simulink model "MdXXIsPosChk"  (R2024b)
settings: Solver=FixedStepDiscrete  StartTime=0.0  StopTime=10.0  FixedStep=0.01  RelTol=1e-3
libraries: simulink x35
(part 2 of 2)

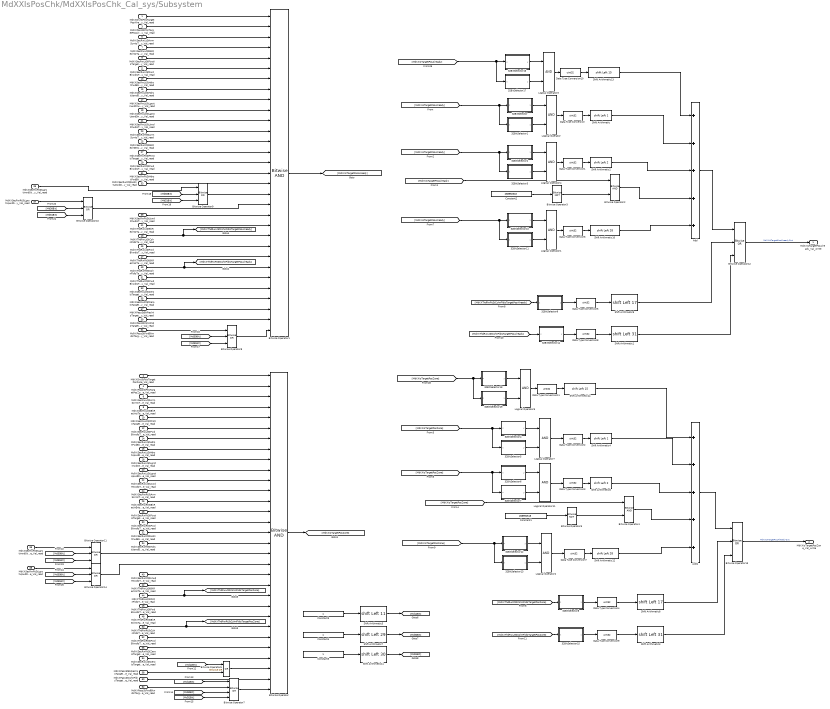
== system MdXXIsPosChk/MdXXIsPosChk_Cal_sys/Subsystem ==
  MdXXDrvStFtIsTargetPosAlready_Val_read : Inport
  MdXXDrvStFtIsTargetPosZone_Val_read : Inport  Port=2
  MdXXPassStFtIsTargetPosAlready_Val_read : Inport  Port=3
  MdXXPassStFtIsTargetPosZone_Val_read : Inport  Port=4
  MdXXSecRwLtStArmScrnIsTargetPosAlready_Val_read : Inport  Port=5
  MdXXSecRwLtStArmScrnIsTargetPosZone_Val_read : Inport  Port=6
  MdXXSecRwLtStBkReclnIsTargetPosAlready_Val_read : Inport  Port=7
  MdXXSecRwLtStBkReclnIsTargetPosZone_Val_read : Inport  Port=8
  MdXXSecRwLtStFtrstIsTargetPosAlready_Val_read : Inport  Port=9
  MdXXSecRwLtStFtrstIsTargetPosZone_Val_read : Inport  Port=10
  MdXXSecRwLtStFwdBkwdIsTargetPosAlready_Val_read : Inport  Port=11
  MdXXSecRwLtStFwdBkwdIsTargetPosZone_Val_read : Inport  Port=12
  MdXXSecRwLtStHdrstFwdBkwdIsTargetPosAlready_Val_read : Inport  Port=13
  MdXXSecRwLtStHdrstFwdBkwdIsTargetPosZone_Val_read : Inport  Port=14
  MdXXSecRwLtStHdrstUpwdDnwdIsTargetPosAlready_Val_read : Inport  Port=15
  MdXXSecRwLtStHdrstUpwdDnwdIsTargetPosZone_Val_read : Inport  Port=16
  MdXXSecRwLtStLgrstInwdOtwdIsTargetPosAlready_Val_read : Inport  Port=17
  MdXXSecRwLtStLgrstInwdOtwdIsTargetPosZone_Val_read : Inport  Port=18
  MdXXSecRwLtStLgrstUpwdDnwdIsTargetPosAlready_Val_read : Inport  Port=19
  MdXXSecRwLtStLgrstUpwdDnwdIsTargetPosZone_Val_read : Inport  Port=20
  MdXXSecRwLtStLtwdRtwdIsTargetPosAlready_Val_read : Inport  Port=21
  MdXXSecRwLtStLtwdRtwdIsTargetPosZone_Val_read : Inport  Port=22
  MdXXSecRwRtStArmScrnIsTargetPosAlready_Val_read : Inport  Port=23
  MdXXSecRwRtStArmScrnIsTargetPosZone_Val_read : Inport  Port=24
  MdXXSecRwRtStBkReclnEnIsTargetPosAlready_Val_read : Inport  Port=25
  MdXXSecRwRtStBkReclnEnIsTargetPosZone_Val_read : Inport  Port=26
  MdXXSecRwRtStFtrstIsTargetPosAlready_Val_read : Inport  Port=27
  MdXXSecRwRtStFtrstIsTargetPosZone_Val_read : Inport  Port=28
  MdXXSecRwRtStFwdBkwdIsTargetPosAlready_Val_read : Inport  Port=29
  MdXXSecRwRtStFwdBkwdIsTargetPosZone_Val_read : Inport  Port=30
  MdXXSecRwRtStHdrstFwdBkwdIsTargetPosAlready_Val_read : Inport  Port=31
  MdXXSecRwRtStHdrstFwdBkwdIsTargetPosZone_Val_read : Inport  Port=32
  MdXXSecRwRtStHdrstUpwdDnwdIsTargetPosAlready_Val_read : Inport  Port=33
  MdXXSecRwRtStHdrstUpwdDnwdIsTargetPosZone_Val_read : Inport  Port=34
  MdXXSecRwRtStLgrstInwdOtwdIsTargetPosAlready_Val_read : Inport  Port=35
  MdXXSecRwRtStLgrstInwdOtwdIsTargetPosZone_Val_read : Inport  Port=36
  MdXXSecRwRtStLgrstUpwdDnwdIsTargetPosAlready_Val_read : Inport  Port=37
  MdXXSecRwRtStLgrstUpwdDnwdIsTargetPosZone_Val_read : Inport  Port=38
  MdXXSecRwRtStLtwdRtwdIsTargetPosAlready_Val_read : Inport  Port=39
  MdXXSecRwRtStLtwdRtwdIsTargetPosZone_Val_read : Inport  Port=40
  MdXXThdRwLtStBkReclnIsTargetPosAlready_Val_read : Inport  Port=41
  MdXXThdRwLtStBkReclnIsTargetPosZone_Val_read : Inport  Port=42
  MdXXThdRwLtStCshnFldIsTargetPosAlready_Val_read : Inport  Port=43
  MdXXThdRwLtStCshnFldIsTargetPosZone_Val_read : Inport  Port=44
  MdXXThdRwLtStFwdBkwdIsTargetPosAlready_Val_read : Inport  Port=45
  MdXXThdRwLtStFwdBkwdIsTargetPosZone_Val_read : Inport  Port=46
  MdXXThdRwRtStBkReclnIsTargetPosAlready_Val_read : Inport  Port=47
  MdXXThdRwRtStBkReclnIsTargetPosZone_Val_read : Inport  Port=48
  MdXXThdRwRtStCshnFldIsTargetPosAlready_Val_read : Inport  Port=49
  MdXXThdRwRtStCshnFldIsTargetPosZone_Val_read : Inport  Port=50
  MdXXThdRwRtStFwdBkwdIsTargetPosAlready_Val_read : Inport  Port=51
  MdXXThdRwRtStFwdBkwdIsTargetPosZone_Val_read : Inport  Port=52
  MdXXSecRwLtStZeroIsTargetPosAlready_Val_read : Inport  Port=53
  MdXXSecRwLtStZeroIsTargetPosZone_Val_read : Inport  Port=54
  MdXXSecRwRtStZeroIsTargetPosAlready_Val_read : Inport  Port=55
  MdXXSecRwRtStZeroIsTargetPosZone_Val_read : Inport  Port=56
  MdXXPassStBkReclnIsTargetPosAlready_Val_read : Inport  Port=57
  MdXXPassStBkReclnIsTargetPosZone_Val_read : Inport  Port=58
  MdXXPassStCshnFldIsTargetPosAlready_Val_read : Inport  Port=59
  MdXXPassStCshnFldIsTargetPosZone_Val_read : Inport  Port=60
  MdXXPassStFwdBkwdIsTargetPosAlready_Val_read : Inport  Port=61
  MdXXPassStFwdBkwdIsTargetPosZone_Val_read : Inport  Port=62
  32BitSelector : Subsystem  mask(32 Bit Selector){BitNum=9}
      mask prompts: BitNum "Select Bit Number"
      mask help: Allows selection of a particular bit (0-31) out of a packed word up to 32 bits long. Output will be true if the bit number selected via the mask parameter is equal to one.
      mask TypeOptions BitNum: 0 | 1 | 2 | 3 | 4 | 5 | 6 | 7 | 8 | 9 | 10 | 11 | 12 | 13 | 14 | 15 | 16 | 17 | 18 | 19 | 20 | 21 | 22 | 23 | 24 | 25 | 26 | 27 | 28 | 29 | 30 | 31
      mask Display:
      | text(0.5, 0.8,'BIT','horizontalAlignment','center')
      | text(0.5, 0.5,'SELECTOR','horizontalAlignment','center')
      | text(0.5, 0.2,['-- Bit ',char(get_param(gcb,'BitNum')),' --'],'horizontalAlignment','center')
  32BitSelector1 : Subsystem  mask(32 Bit Selector){BitNum=11}
      mask prompts: BitNum "Select Bit Number"
      mask help: Allows selection of a particular bit (0-31) out of a packed word up to 32 bits long. Output will be true if the bit number selected via the mask parameter is equal to one.
      mask TypeOptions BitNum: 0 | 1 | 2 | 3 | 4 | 5 | 6 | 7 | 8 | 9 | 10 | 11 | 12 | 13 | 14 | 15 | 16 | 17 | 18 | 19 | 20 | 21 | 22 | 23 | 24 | 25 | 26 | 27 | 28 | 29 | 30 | 31
      mask Display:
      | text(0.5, 0.8,'BIT','horizontalAlignment','center')
      | text(0.5, 0.5,'SELECTOR','horizontalAlignment','center')
      | text(0.5, 0.2,['-- Bit ',char(get_param(gcb,'BitNum')),' --'],'horizontalAlignment','center')
  32BitSelector10 : Subsystem  mask(32 Bit Selector){BitNum=26}
      mask prompts: BitNum "Select Bit Number"
      mask help: Allows selection of a particular bit (0-31) out of a packed word up to 32 bits long. Output will be true if the bit number selected via the mask parameter is equal to one.
      mask TypeOptions BitNum: 0 | 1 | 2 | 3 | 4 | 5 | 6 | 7 | 8 | 9 | 10 | 11 | 12 | 13 | 14 | 15 | 16 | 17 | 18 | 19 | 20 | 21 | 22 | 23 | 24 | 25 | 26 | 27 | 28 | 29 | 30 | 31
      mask Display:
      | text(0.5, 0.8,'BIT','horizontalAlignment','center')
      | text(0.5, 0.5,'SELECTOR','horizontalAlignment','center')
      | text(0.5, 0.2,['-- Bit ',char(get_param(gcb,'BitNum')),' --'],'horizontalAlignment','center')
  32BitSelector11 : Subsystem  mask(32 Bit Selector){BitNum=27}
      mask prompts: BitNum "Select Bit Number"
      mask help: Allows selection of a particular bit (0-31) out of a packed word up to 32 bits long. Output will be true if the bit number selected via the mask parameter is equal to one.
      mask TypeOptions BitNum: 0 | 1 | 2 | 3 | 4 | 5 | 6 | 7 | 8 | 9 | 10 | 11 | 12 | 13 | 14 | 15 | 16 | 17 | 18 | 19 | 20 | 21 | 22 | 23 | 24 | 25 | 26 | 27 | 28 | 29 | 30 | 31
      mask Display:
      | text(0.5, 0.8,'BIT','horizontalAlignment','center')
      | text(0.5, 0.5,'SELECTOR','horizontalAlignment','center')
      | text(0.5, 0.2,['-- Bit ',char(get_param(gcb,'BitNum')),' --'],'horizontalAlignment','center')
  32BitSelector12 : Subsystem  mask(32 Bit Selector){BitNum=26}
      mask prompts: BitNum "Select Bit Number"
      mask help: Allows selection of a particular bit (0-31) out of a packed word up to 32 bits long. Output will be true if the bit number selected via the mask parameter is equal to one.
      mask TypeOptions BitNum: 0 | 1 | 2 | 3 | 4 | 5 | 6 | 7 | 8 | 9 | 10 | 11 | 12 | 13 | 14 | 15 | 16 | 17 | 18 | 19 | 20 | 21 | 22 | 23 | 24 | 25 | 26 | 27 | 28 | 29 | 30 | 31
      mask Display:
      | text(0.5, 0.8,'BIT','horizontalAlignment','center')
      | text(0.5, 0.5,'SELECTOR','horizontalAlignment','center')
      | text(0.5, 0.2,['-- Bit ',char(get_param(gcb,'BitNum')),' --'],'horizontalAlignment','center')
  32BitSelector13 : Subsystem  mask(32 Bit Selector){BitNum=27}
      mask prompts: BitNum "Select Bit Number"
      mask help: Allows selection of a particular bit (0-31) out of a packed word up to 32 bits long. Output will be true if the bit number selected via the mask parameter is equal to one.
      mask TypeOptions BitNum: 0 | 1 | 2 | 3 | 4 | 5 | 6 | 7 | 8 | 9 | 10 | 11 | 12 | 13 | 14 | 15 | 16 | 17 | 18 | 19 | 20 | 21 | 22 | 23 | 24 | 25 | 26 | 27 | 28 | 29 | 30 | 31
      mask Display:
      | text(0.5, 0.8,'BIT','horizontalAlignment','center')
      | text(0.5, 0.5,'SELECTOR','horizontalAlignment','center')
      | text(0.5, 0.2,['-- Bit ',char(get_param(gcb,'BitNum')),' --'],'horizontalAlignment','center')
  32BitSelector14 : Subsystem  mask(32 Bit Selector){BitNum=31}
      mask prompts: BitNum "Select Bit Number"
      mask help: Allows selection of a particular bit (0-31) out of a packed word up to 32 bits long. Output will be true if the bit number selected via the mask parameter is equal to one.
      mask TypeOptions BitNum: 0 | 1 | 2 | 3 | 4 | 5 | 6 | 7 | 8 | 9 | 10 | 11 | 12 | 13 | 14 | 15 | 16 | 17 | 18 | 19 | 20 | 21 | 22 | 23 | 24 | 25 | 26 | 27 | 28 | 29 | 30 | 31
      mask Display:
      | text(0.5, 0.8,'BIT','horizontalAlignment','center')
      | text(0.5, 0.5,'SELECTOR','horizontalAlignment','center')
      | text(0.5, 0.2,['-- Bit ',char(get_param(gcb,'BitNum')),' --'],'horizontalAlignment','center')
  32BitSelector15 : Subsystem  mask(32 Bit Selector){BitNum=31}
      mask prompts: BitNum "Select Bit Number"
      mask help: Allows selection of a particular bit (0-31) out of a packed word up to 32 bits long. Output will be true if the bit number selected via the mask parameter is equal to one.
      mask TypeOptions BitNum: 0 | 1 | 2 | 3 | 4 | 5 | 6 | 7 | 8 | 9 | 10 | 11 | 12 | 13 | 14 | 15 | 16 | 17 | 18 | 19 | 20 | 21 | 22 | 23 | 24 | 25 | 26 | 27 | 28 | 29 | 30 | 31
      mask Display:
      | text(0.5, 0.8,'BIT','horizontalAlignment','center')
      | text(0.5, 0.5,'SELECTOR','horizontalAlignment','center')
      | text(0.5, 0.2,['-- Bit ',char(get_param(gcb,'BitNum')),' --'],'horizontalAlignment','center')
  32BitSelector16 : Subsystem  mask(32 Bit Selector){BitNum=13}
      mask prompts: BitNum "Select Bit Number"
      mask help: Allows selection of a particular bit (0-31) out of a packed word up to 32 bits long. Output will be true if the bit number selected via the mask parameter is equal to one.
      mask TypeOptions BitNum: 0 | 1 | 2 | 3 | 4 | 5 | 6 | 7 | 8 | 9 | 10 | 11 | 12 | 13 | 14 | 15 | 16 | 17 | 18 | 19 | 20 | 21 | 22 | 23 | 24 | 25 | 26 | 27 | 28 | 29 | 30 | 31
      mask Display:
      | text(0.5, 0.8,'BIT','horizontalAlignment','center')
      | text(0.5, 0.5,'SELECTOR','horizontalAlignment','center')
      | text(0.5, 0.2,['-- Bit ',char(get_param(gcb,'BitNum')),' --'],'horizontalAlignment','center')
  32BitSelector17 : Subsystem  mask(32 Bit Selector){BitNum=14}
      mask prompts: BitNum "Select Bit Number"
      mask help: Allows selection of a particular bit (0-31) out of a packed word up to 32 bits long. Output will be true if the bit number selected via the mask parameter is equal to one.
      mask TypeOptions BitNum: 0 | 1 | 2 | 3 | 4 | 5 | 6 | 7 | 8 | 9 | 10 | 11 | 12 | 13 | 14 | 15 | 16 | 17 | 18 | 19 | 20 | 21 | 22 | 23 | 24 | 25 | 26 | 27 | 28 | 29 | 30 | 31
      mask Display:
      | text(0.5, 0.8,'BIT','horizontalAlignment','center')
      | text(0.5, 0.5,'SELECTOR','horizontalAlignment','center')
      | text(0.5, 0.2,['-- Bit ',char(get_param(gcb,'BitNum')),' --'],'horizontalAlignment','center')
  32BitSelector18 : Subsystem  mask(32 Bit Selector){BitNum=13}
      mask prompts: BitNum "Select Bit Number"
      mask help: Allows selection of a particular bit (0-31) out of a packed word up to 32 bits long. Output will be true if the bit number selected via the mask parameter is equal to one.
      mask TypeOptions BitNum: 0 | 1 | 2 | 3 | 4 | 5 | 6 | 7 | 8 | 9 | 10 | 11 | 12 | 13 | 14 | 15 | 16 | 17 | 18 | 19 | 20 | 21 | 22 | 23 | 24 | 25 | 26 | 27 | 28 | 29 | 30 | 31
      mask Display:
      | text(0.5, 0.8,'BIT','horizontalAlignment','center')
      | text(0.5, 0.5,'SELECTOR','horizontalAlignment','center')
      | text(0.5, 0.2,['-- Bit ',char(get_param(gcb,'BitNum')),' --'],'horizontalAlignment','center')
  32BitSelector19 : Subsystem  mask(32 Bit Selector){BitNum=14}
      mask prompts: BitNum "Select Bit Number"
      mask help: Allows selection of a particular bit (0-31) out of a packed word up to 32 bits long. Output will be true if the bit number selected via the mask parameter is equal to one.
      mask TypeOptions BitNum: 0 | 1 | 2 | 3 | 4 | 5 | 6 | 7 | 8 | 9 | 10 | 11 | 12 | 13 | 14 | 15 | 16 | 17 | 18 | 19 | 20 | 21 | 22 | 23 | 24 | 25 | 26 | 27 | 28 | 29 | 30 | 31
      mask Display:
      | text(0.5, 0.8,'BIT','horizontalAlignment','center')
      | text(0.5, 0.5,'SELECTOR','horizontalAlignment','center')
      | text(0.5, 0.2,['-- Bit ',char(get_param(gcb,'BitNum')),' --'],'horizontalAlignment','center')
  32BitSelector2 : Subsystem  mask(32 Bit Selector){BitNum=7}
      mask prompts: BitNum "Select Bit Number"
      mask help: Allows selection of a particular bit (0-31) out of a packed word up to 32 bits long. Output will be true if the bit number selected via the mask parameter is equal to one.
      mask TypeOptions BitNum: 0 | 1 | 2 | 3 | 4 | 5 | 6 | 7 | 8 | 9 | 10 | 11 | 12 | 13 | 14 | 15 | 16 | 17 | 18 | 19 | 20 | 21 | 22 | 23 | 24 | 25 | 26 | 27 | 28 | 29 | 30 | 31
      mask Display:
      | text(0.5, 0.8,'BIT','horizontalAlignment','center')
      | text(0.5, 0.5,'SELECTOR','horizontalAlignment','center')
      | text(0.5, 0.2,['-- Bit ',char(get_param(gcb,'BitNum')),' --'],'horizontalAlignment','center')
  32BitSelector3 : Subsystem  mask(32 Bit Selector){BitNum=8}
      mask prompts: BitNum "Select Bit Number"
      mask help: Allows selection of a particular bit (0-31) out of a packed word up to 32 bits long. Output will be true if the bit number selected via the mask parameter is equal to one.
      mask TypeOptions BitNum: 0 | 1 | 2 | 3 | 4 | 5 | 6 | 7 | 8 | 9 | 10 | 11 | 12 | 13 | 14 | 15 | 16 | 17 | 18 | 19 | 20 | 21 | 22 | 23 | 24 | 25 | 26 | 27 | 28 | 29 | 30 | 31
      mask Display:
      | text(0.5, 0.8,'BIT','horizontalAlignment','center')
      | text(0.5, 0.5,'SELECTOR','horizontalAlignment','center')
      | text(0.5, 0.2,['-- Bit ',char(get_param(gcb,'BitNum')),' --'],'horizontalAlignment','center')
  32BitSelector4 : Subsystem  mask(32 Bit Selector){BitNum=9}
      mask prompts: BitNum "Select Bit Number"
      mask help: Allows selection of a particular bit (0-31) out of a packed word up to 32 bits long. Output will be true if the bit number selected via the mask parameter is equal to one.
      mask TypeOptions BitNum: 0 | 1 | 2 | 3 | 4 | 5 | 6 | 7 | 8 | 9 | 10 | 11 | 12 | 13 | 14 | 15 | 16 | 17 | 18 | 19 | 20 | 21 | 22 | 23 | 24 | 25 | 26 | 27 | 28 | 29 | 30 | 31
      mask Display:
      | text(0.5, 0.8,'BIT','horizontalAlignment','center')
      | text(0.5, 0.5,'SELECTOR','horizontalAlignment','center')
      | text(0.5, 0.2,['-- Bit ',char(get_param(gcb,'BitNum')),' --'],'horizontalAlignment','center')
  32BitSelector5 : Subsystem  mask(32 Bit Selector){BitNum=11}
      mask prompts: BitNum "Select Bit Number"
      mask help: Allows selection of a particular bit (0-31) out of a packed word up to 32 bits long. Output will be true if the bit number selected via the mask parameter is equal to one.
      mask TypeOptions BitNum: 0 | 1 | 2 | 3 | 4 | 5 | 6 | 7 | 8 | 9 | 10 | 11 | 12 | 13 | 14 | 15 | 16 | 17 | 18 | 19 | 20 | 21 | 22 | 23 | 24 | 25 | 26 | 27 | 28 | 29 | 30 | 31
      mask Display:
      | text(0.5, 0.8,'BIT','horizontalAlignment','center')
      | text(0.5, 0.5,'SELECTOR','horizontalAlignment','center')
      | text(0.5, 0.2,['-- Bit ',char(get_param(gcb,'BitNum')),' --'],'horizontalAlignment','center')
  32BitSelector6 : Subsystem  mask(32 Bit Selector){BitNum=7}
      mask prompts: BitNum "Select Bit Number"
      mask help: Allows selection of a particular bit (0-31) out of a packed word up to 32 bits long. Output will be true if the bit number selected via the mask parameter is equal to one.
      mask TypeOptions BitNum: 0 | 1 | 2 | 3 | 4 | 5 | 6 | 7 | 8 | 9 | 10 | 11 | 12 | 13 | 14 | 15 | 16 | 17 | 18 | 19 | 20 | 21 | 22 | 23 | 24 | 25 | 26 | 27 | 28 | 29 | 30 | 31
      mask Display:
      | text(0.5, 0.8,'BIT','horizontalAlignment','center')
      | text(0.5, 0.5,'SELECTOR','horizontalAlignment','center')
      | text(0.5, 0.2,['-- Bit ',char(get_param(gcb,'BitNum')),' --'],'horizontalAlignment','center')
  32BitSelector7 : Subsystem  mask(32 Bit Selector){BitNum=8}
      mask prompts: BitNum "Select Bit Number"
      mask help: Allows selection of a particular bit (0-31) out of a packed word up to 32 bits long. Output will be true if the bit number selected via the mask parameter is equal to one.
      mask TypeOptions BitNum: 0 | 1 | 2 | 3 | 4 | 5 | 6 | 7 | 8 | 9 | 10 | 11 | 12 | 13 | 14 | 15 | 16 | 17 | 18 | 19 | 20 | 21 | 22 | 23 | 24 | 25 | 26 | 27 | 28 | 29 | 30 | 31
      mask Display:
      | text(0.5, 0.8,'BIT','horizontalAlignment','center')
      | text(0.5, 0.5,'SELECTOR','horizontalAlignment','center')
      | text(0.5, 0.2,['-- Bit ',char(get_param(gcb,'BitNum')),' --'],'horizontalAlignment','center')
  32BitSelector8 : Subsystem  mask(32 Bit Selector){BitNum=17}
      mask prompts: BitNum "Select Bit Number"
      mask help: Allows selection of a particular bit (0-31) out of a packed word up to 32 bits long. Output will be true if the bit number selected via the mask parameter is equal to one.
      mask TypeOptions BitNum: 0 | 1 | 2 | 3 | 4 | 5 | 6 | 7 | 8 | 9 | 10 | 11 | 12 | 13 | 14 | 15 | 16 | 17 | 18 | 19 | 20 | 21 | 22 | 23 | 24 | 25 | 26 | 27 | 28 | 29 | 30 | 31
      mask Display:
      | text(0.5, 0.8,'BIT','horizontalAlignment','center')
      | text(0.5, 0.5,'SELECTOR','horizontalAlignment','center')
      | text(0.5, 0.2,['-- Bit ',char(get_param(gcb,'BitNum')),' --'],'horizontalAlignment','center')
  32BitSelector9 : Subsystem  mask(32 Bit Selector){BitNum=17}
      mask prompts: BitNum "Select Bit Number"
      mask help: Allows selection of a particular bit (0-31) out of a packed word up to 32 bits long. Output will be true if the bit number selected via the mask parameter is equal to one.
      mask TypeOptions BitNum: 0 | 1 | 2 | 3 | 4 | 5 | 6 | 7 | 8 | 9 | 10 | 11 | 12 | 13 | 14 | 15 | 16 | 17 | 18 | 19 | 20 | 21 | 22 | 23 | 24 | 25 | 26 | 27 | 28 | 29 | 30 | 31
      mask Display:
      | text(0.5, 0.8,'BIT','horizontalAlignment','center')
      | text(0.5, 0.5,'SELECTOR','horizontalAlignment','center')
      | text(0.5, 0.2,['-- Bit ',char(get_param(gcb,'BitNum')),' --'],'horizontalAlignment','center')
  Add : Sum  Inputs=+++++  OutDataTypeStr=uint32
  Add1 : Sum  Inputs=+++++  AccumDataTypeStr=uint32
  Bitwise Operator : simulink/Logic and Bit Operations/Bitwise Operator  logicop=AND  UseBitMask=off  NumInputPorts=31  BitMask=bin2dec('11011001')  BitMaskRealWorld=Stored Integer
  Bitwise Operator1 : simulink/Logic and Bit Operations/Bitwise Operator  logicop=AND  UseBitMask=off  NumInputPorts=31  BitMask=bin2dec('11011001')  BitMaskRealWorld=Stored Integer
  Bitwise Operator{8..14} (7 alike) : simulink/Logic and Bit Operations/Bitwise Operator  logicop=OR  UseBitMask=off  NumInputPorts=3  BitMask=bin2dec('11011001')  BitMaskRealWorld=Stored Integer
  Bitwise Operator2 : simulink/Logic and Bit Operations/Bitwise Operator  logicop=AND  UseBitMask=off  NumInputPorts=2  BitMask=bin2dec('11011001')  BitMaskRealWorld=Stored Integer
  Bitwise Operator3 : simulink/Logic and Bit Operations/Bitwise Operator  logicop=NOT  UseBitMask=off  BitMask=bin2dec('11011001')  BitMaskRealWorld=Stored Integer
  Bitwise Operator4 : simulink/Logic and Bit Operations/Bitwise Operator  logicop=AND  UseBitMask=off  NumInputPorts=2  BitMask=bin2dec('11011001')  BitMaskRealWorld=Stored Integer
  Bitwise Operator5 : simulink/Logic and Bit Operations/Bitwise Operator  logicop=NOT  UseBitMask=off  BitMask=bin2dec('11011001')  BitMaskRealWorld=Stored Integer
  Bitwise Operator6 : simulink/Logic and Bit Operations/Bitwise Operator  logicop=OR  UseBitMask=off  NumInputPorts=2  BitMask=bin2dec('11011001')  BitMaskRealWorld=Stored Integer
  Bitwise Operator7 : simulink/Logic and Bit Operations/Bitwise Operator  logicop=OR  UseBitMask=off  NumInputPorts=4  BitMask=bin2dec('11011001')  BitMaskRealWorld=Stored Integer
  Constant1 : Constant  Value=268992518  OutDataTypeStr=uint32
  Constant2 : Constant  Value=268992518  OutDataTypeStr=uint32
  Constant3 : Constant  OutDataTypeStr=uint32
  Constant4 : Constant  OutDataTypeStr=uint32
  Constant5 : Constant  OutDataTypeStr=uint32
  Data Type Conversion{,1..11} (12 alike) : DataTypeConversion  OutDataTypeStr=uint32  SaturateOnIntegerOverflow=off  RndMeth=Floor
  Logical Operator{,1..5,7,11} (8 alike) : Logic  AllPortsSameDT=off  OutDataTypeStr=boolean
  Shift Arithmetic : ArithShift  BitShiftNumber=1  BitShiftDirection=Left
  Shift Arithmetic1 : ArithShift  BitShiftNumber=31  BitShiftDirection=Left
  Shift Arithmetic10 : ArithShift  BitShiftNumber=28  BitShiftDirection=Left
  Shift Arithmetic11 : ArithShift  BitShiftNumber=30  BitShiftDirection=Left
  Shift Arithmetic12 : ArithShift  BitShiftNumber=28  BitShiftDirection=Left
  Shift Arithmetic13 : ArithShift  BitShiftNumber=15  BitShiftDirection=Left
  Shift Arithmetic14 : ArithShift  BitShiftNumber=15  BitShiftDirection=Left
  Shift Arithmetic2 : ArithShift  BitShiftNumber=2  BitShiftDirection=Left
  Shift Arithmetic3 : ArithShift  BitShiftNumber=31  BitShiftDirection=Left
  Shift Arithmetic4 : ArithShift  BitShiftNumber=1  BitShiftDirection=Left
  Shift Arithmetic5 : ArithShift  BitShiftNumber=11  BitShiftDirection=Left
  Shift Arithmetic6 : ArithShift  BitShiftNumber=2  BitShiftDirection=Left
  Shift Arithmetic7 : ArithShift  BitShiftNumber=29  BitShiftDirection=Left
  Shift Arithmetic8 : ArithShift  BitShiftNumber=17  BitShiftDirection=Left
  Shift Arithmetic9 : ArithShift  BitShiftNumber=17  BitShiftDirection=Left
  MdXXIsTargetPosAlready_Val_write : Outport  VectorParamsAs1DForOutWhenUnconnected=off
      settings: EnsureOutportIsVirtual=on
  MdXXIsTargetPosZone_Val_write : Outport  Port=2  VectorParamsAs1DForOutWhenUnconnected=off
      settings: EnsureOutportIsVirtual=on
  wires:
  MdXXThdRwRtStBkReclnIsTargetPosAlready_Val_read/1 -> Bitwise Operator1/24
  MdXXThdRwLtStFwdBkwdIsTargetPosAlready_Val_read/1 -> Bitwise Operator1/23
  MdXXThdRwLtStBkReclnIsTargetPosAlready_Val_read/1 -> Bitwise Operator1/21
  MdXXThdRwLtStCshnFldIsTargetPosAlready_Val_read/1 -> [MdXXThdRwLtStCshnFldIsTargetPosAlready], Bitwise Operator1/22
  MdXXThdRwRtStCshnFldIsTargetPosAlready_Val_read/1 -> [MdXXThdRwRtStCshnFldIsTargetPosAlready], Bitwise Operator1/25
  MdXXSecRwLtStLtwdRtwdIsTargetPosAlready_Val_read/1 -> Bitwise Operator1/11
  MdXXSecRwRtStArmScrnIsTargetPosAlready_Val_read/1 -> Bitwise Operator1/12
  MdXXSecRwRtStBkReclnEnIsTargetPosAlready_Val_read/1 -> Bitwise Operator1/13
  MdXXSecRwRtStFwdBkwdIsTargetPosAlready_Val_read/1 -> Bitwise Operator1/15
  MdXXSecRwRtStHdrstFwdBkwdIsTargetPosAlready_Val_read/1 -> Bitwise Operator1/16
  MdXXSecRwRtStHdrstUpwdDnwdIsTargetPosAlready_Val_read/1 -> Bitwise Operator1/17
  MdXXSecRwRtStLtwdRtwdIsTargetPosAlready_Val_read/1 -> Bitwise Operator1/20
  MdXXThdRwRtStFwdBkwdIsTargetPosAlready_Val_read/1 -> Bitwise Operator1/26
  MdXXSecRwLtStLgrstUpwdDnwdIsTargetPosAlready_Val_read/1 -> Bitwise Operator1/10
  MdXXSecRwRtStFtrstIsTargetPosAlready_Val_read/1 -> Bitwise Operator1/14
  MdXXSecRwLtStHdrstUpwdDnwdIsTargetPosAlready_Val_read/1 -> Bitwise Operator1/8
  MdXXSecRwLtStLgrstInwdOtwdIsTargetPosAlready_Val_read/1 -> Bitwise Operator1/9
  MdXXSecRwLtStFtrstIsTargetPosAlready_Val_read/1 -> Bitwise Operator1/5
  MdXXSecRwLtStFwdBkwdIsTargetPosAlready_Val_read/1 -> Bitwise Operator1/6
  MdXXSecRwLtStHdrstFwdBkwdIsTargetPosAlready_Val_read/1 -> Bitwise Operator1/7
  MdXXDrvStFtIsTargetPosAlready_Val_read/1 -> Bitwise Operator1/1
  MdXXPassStFtIsTargetPosAlready_Val_read/1 -> Bitwise Operator1/2
  MdXXSecRwLtStArmScrnIsTargetPosAlready_Val_read/1 -> Bitwise Operator1/3
  MdXXSecRwLtStBkReclnIsTargetPosAlready_Val_read/1 -> Bitwise Operator1/4
  MdXXThdRwRtStFwdBkwdIsTargetPosZone_Val_read/1 -> Bitwise Operator/26
  MdXXThdRwRtStCshnFldIsTargetPosZone_Val_read/1 -> [MdXXThdRwRtStCshnFldIsTargetPosZone], Bitwise Operator/25
  MdXXThdRwRtStBkReclnIsTargetPosZone_Val_read/1 -> Bitwise Operator/24
  MdXXThdRwLtStFwdBkwdIsTargetPosZone_Val_read/1 -> Bitwise Operator/23
  MdXXThdRwLtStCshnFldIsTargetPosZone_Val_read/1 -> [MdXXThdRwLtStCshnFldIsTargetPosZone], Bitwise Operator/22
  MdXXThdRwLtStBkReclnIsTargetPosZone_Val_read/1 -> Bitwise Operator/21
  MdXXSecRwRtStLtwdRtwdIsTargetPosZone_Val_read/1 -> Bitwise Operator/20
  MdXXSecRwRtStHdrstUpwdDnwdIsTargetPosZone_Val_read/1 -> Bitwise Operator/17
  MdXXSecRwRtStHdrstFwdBkwdIsTargetPosZone_Val_read/1 -> Bitwise Operator/16
  MdXXSecRwRtStFwdBkwdIsTargetPosZone_Val_read/1 -> Bitwise Operator/15
  MdXXSecRwRtStFtrstIsTargetPosZone_Val_read/1 -> Bitwise Operator/14
  MdXXSecRwRtStBkReclnEnIsTargetPosZone_Val_read/1 -> Bitwise Operator/13
  MdXXSecRwRtStArmScrnIsTargetPosZone_Val_read/1 -> Bitwise Operator/12
  MdXXSecRwLtStLtwdRtwdIsTargetPosZone_Val_read/1 -> Bitwise Operator/11
  MdXXSecRwLtStLgrstUpwdDnwdIsTargetPosZone_Val_read/1 -> Bitwise Operator/10
  MdXXSecRwLtStLgrstInwdOtwdIsTargetPosZone_Val_read/1 -> Bitwise Operator/9
  MdXXSecRwLtStHdrstUpwdDnwdIsTargetPosZone_Val_read/1 -> Bitwise Operator/8
  MdXXSecRwLtStHdrstFwdBkwdIsTargetPosZone_Val_read/1 -> Bitwise Operator/7
  MdXXSecRwLtStFwdBkwdIsTargetPosZone_Val_read/1 -> Bitwise Operator/6
  MdXXSecRwLtStFtrstIsTargetPosZone_Val_read/1 -> Bitwise Operator/5
  MdXXSecRwLtStBkReclnIsTargetPosZone_Val_read/1 -> Bitwise Operator/4
  MdXXSecRwLtStArmScrnIsTargetPosZone_Val_read/1 -> Bitwise Operator/3
  MdXXPassStFtIsTargetPosZone_Val_read/1 -> Bitwise Operator/2
  MdXXDrvStFtIsTargetPosZone_Val_read/1 -> Bitwise Operator/1
  Bitwise Operator1/1 -> [MdXXIsTargetPosAlready]
  [MdXXIsTargetPosAlready] -> 32BitSelector1/1(x), 32BitSelector/1(x)
  32BitSelector/1(y) -> Logical Operator/1
  32BitSelector1/1(y) -> Logical Operator/2
  Logical Operator/1 -> Data Type Conversion/1
  Shift Arithmetic/1 -> Add/2
  Data Type Conversion/1 -> Shift Arithmetic/1
  Bitwise Operator12/1 -> MdXXIsTargetPosAlready_Val_write/1  "MdXXIsTargetPosAlreadyOut"
  32BitSelector3/1(y) -> Logical Operator4/2
  32BitSelector2/1(y) -> Logical Operator4/1
  [MdXXIsTargetPosAlready] -> 32BitSelector2/1(x), 32BitSelector3/1(x)
  Data Type Conversion1/1 -> Shift Arithmetic2/1
  Shift Arithmetic2/1 -> Add/3
  Logical Operator4/1 -> Data Type Conversion1/1
  Logical Operator11/1 -> Data Type Conversion3/1
  Shift Arithmetic6/1 -> Add1/3
  Data Type Conversion3/1 -> Shift Arithmetic6/1
  [MdXXIsTargetPosZone] -> 32BitSelector7/1(x), 32BitSelector6/1(x)
  32BitSelector6/1(y) -> Logical Operator11/1
  32BitSelector7/1(y) -> Logical Operator11/2
  Data Type Conversion2/1 -> Shift Arithmetic4/1
  Shift Arithmetic4/1 -> Add1/2
  Logical Operator7/1 -> Data Type Conversion2/1
  32BitSelector5/1(y) -> Logical Operator7/2
  32BitSelector4/1(y) -> Logical Operator7/1
  [MdXXIsTargetPosZone] -> 32BitSelector4/1(x), 32BitSelector5/1(x)
  Bitwise Operator/1 -> [MdXXIsTargetPosZone]
  MdXXSecRwLtStZeroIsTargetPosAlready_Val_read/1 -> Bitwise Operator1/27
  MdXXSecRwRtStZeroIsTargetPosAlready_Val_read/1 -> Bitwise Operator1/28
  MdXXPassStBkReclnIsTargetPosAlready_Val_read/1 -> Bitwise Operator1/29
  MdXXPassStCshnFldIsTargetPosAlready_Val_read/1 -> Bitwise Operator1/30
  [MdXXThdRwRtStCshnFldIsTargetPosZone] -> 32BitSelector8/1(x)
  32BitSelector8/1(y) -> Data Type Conversion4/1
  Data Type Conversion4/1 -> Shift Arithmetic8/1
  Shift Arithmetic8/1 -> Bitwise Operator13/2
  Data Type Conversion5/1 -> Shift Arithmetic9/1
  32BitSelector9/1(y) -> Data Type Conversion5/1
  [MdXXThdRwRtStCshnFldIsTargetPosAlready] -> 32BitSelector9/1(x)
  MdXXSecRwRtStZeroIsTargetPosZone_Val_read/1 -> Bitwise Operator/27
  MdXXSecRwLtStZeroIsTargetPosZone_Val_read/1 -> Bitwise Operator/28
  MdXXPassStCshnFldIsTargetPosZone_Val_read/1 -> Bitwise Operator/30
  Shift Arithmetic9/1 -> Bitwise Operator12/2
  Add/1 -> Bitwise Operator12/1
  Add1/1 -> Bitwise Operator13/1
  Bitwise Operator13/1 -> MdXXIsTargetPosZone_Val_write/1  "MdXXIsTargetPosAlreadyOut"
  Data Type Conversion6/1 -> Shift Arithmetic10/1
  Shift Arithmetic10/1 -> Add/5
  Logical Operator1/1 -> Data Type Conversion6/1
  32BitSelector10/1(y) -> Logical Operator1/1
  [MdXXIsTargetPosAlready] -> 32BitSelector10/1(x), 32BitSelector11/1(x)
  32BitSelector11/1(y) -> Logical Operator1/2
  Shift Arithmetic12/1 -> Add1/5
  [MdXXIsTargetPosZone] -> 32BitSelector12/1(x), 32BitSelector13/1(x)
  32BitSelector12/1(y) -> Logical Operator2/1
  Data Type Conversion7/1 -> Shift Arithmetic12/1
  32BitSelector13/1(y) -> Logical Operator2/2
  Logical Operator2/1 -> Data Type Conversion7/1
  Bitwise Operator2/1 -> Add/4
  [MdXXIsTargetPosAlready] -> Bitwise Operator2/1
  Bitwise Operator3/1 -> Bitwise Operator2/2
  Constant2/1 -> Bitwise Operator3/1
  Constant1/1 -> Bitwise Operator5/1
  Bitwise Operator5/1 -> Bitwise Operator4/2
  [MdXXIsTargetPosZone] -> Bitwise Operator4/1
  Bitwise Operator4/1 -> Add1/4
  [MdXXThdRwLtStCshnFldIsTargetPosAlready] -> 32BitSelector14/1(x)
  32BitSelector14/1(y) -> Data Type Conversion8/1
  Data Type Conversion8/1 -> Shift Arithmetic1/1
  Shift Arithmetic1/1 -> Bitwise Operator12/3
  [MdXXThdRwLtStCshnFldIsTargetPosZone] -> 32BitSelector15/1(x)
  32BitSelector15/1(y) -> Data Type Conversion9/1
  Data Type Conversion9/1 -> Shift Arithmetic3/1
  Shift Arithmetic3/1 -> Bitwise Operator13/3
  Constant3/1 -> Shift Arithmetic5/1
  Shift Arithmetic5/1 -> [Md12Bit]
  [Md12Bit] -> Bitwise Operator6/1
  MdXXPassStBkReclnIsTargetPosZone_Val_read/1 -> Bitwise Operator6/2
  Bitwise Operator6/1 -> Bitwise Operator/29
  Bitwise Operator7/1 -> Bitwise Operator/31
  [Md12Bit] -> Bitwise Operator7/1
  MdXXPassStFwdBkwdIsTargetPosZone_Val_read/1 -> Bitwise Operator7/2
  [Md30Bit] -> Bitwise Operator7/3
  [Md31Bit] -> Bitwise Operator7/4
  Shift Arithmetic7/1 -> [Md30Bit]
  Constant4/1 -> Shift Arithmetic7/1
  Constant5/1 -> Shift Arithmetic11/1
  Shift Arithmetic11/1 -> [Md31Bit]
  [Md31Bit] -> Bitwise Operator8/3
  [Md30Bit] -> Bitwise Operator8/2
  Bitwise Operator8/1 -> Bitwise Operator1/31
  MdXXPassStFwdBkwdIsTargetPosAlready_Val_read/1 -> Bitwise Operator8/1
  MdXXSecRwRtStLgrstInwdOtwdIsTargetPosAlready_Val_read/1 -> Bitwise Operator9/1
  Bitwise Operator9/1 -> Bitwise Operator1/18
  Bitwise Operator10/1 -> Bitwise Operator1/19
  MdXXSecRwRtStLgrstUpwdDnwdIsTargetPosAlready_Val_read/1 -> Bitwise Operator10/1
  [Md30Bit] -> Bitwise Operator9/2
  [Md31Bit] -> Bitwise Operator9/3
  [Md31Bit] -> Bitwise Operator10/3
  [Md30Bit] -> Bitwise Operator10/2
  Bitwise Operator11/1 -> Bitwise Operator/18
  MdXXSecRwRtStLgrstInwdOtwdIsTargetPosZone_Val_read/1 -> Bitwise Operator11/1
  MdXXSecRwRtStLgrstUpwdDnwdIsTargetPosZone_Val_read/1 -> Bitwise Operator14/1
  Bitwise Operator14/1 -> Bitwise Operator/19
  [Md31Bit] -> Bitwise Operator11/3
  [Md30Bit] -> Bitwise Operator11/2
  [Md31Bit] -> Bitwise Operator14/3
  [Md30Bit] -> Bitwise Operator14/2
  [MdXXIsTargetPosAlready] -> 32BitSelector17/1(x), 32BitSelector16/1(x)
  Data Type Conversion10/1 -> Shift Arithmetic13/1
  32BitSelector17/1(y) -> Logical Operator3/2
  Logical Operator3/1 -> Data Type Conversion10/1
  32BitSelector16/1(y) -> Logical Operator3/1
  Shift Arithmetic13/1 -> Add/1
  [MdXXIsTargetPosZone] -> 32BitSelector19/1(x), 32BitSelector18/1(x)
  32BitSelector18/1(y) -> Logical Operator5/1
  Logical Operator5/1 -> Data Type Conversion11/1
  Data Type Conversion11/1 -> Shift Arithmetic14/1
  Shift Arithmetic14/1 -> Add1/1
  32BitSelector19/1(y) -> Logical Operator5/2

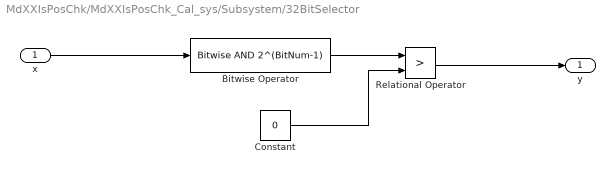
== system MdXXIsPosChk/MdXXIsPosChk_Cal_sys/Subsystem/32BitSelector ==
  x : Inport
  Bitwise Operator : simulink/Logic and Bit Operations/Bitwise Operator  logicop=AND  UseBitMask=on  BitMask=2^(BitNum-1)  BitMaskRealWorld=Stored Integer
  Constant : Constant  Value=0  OutDataTypeStr=uint32
  Relational Operator : RelationalOperator  Operator=>  OutDataTypeStr=boolean  RndMeth=Simplest  InputSameDT=off
  y : Outport  VectorParamsAs1DForOutWhenUnconnected=off
  wires:
  Relational Operator/1 -> y/1
  Constant/1 -> Relational Operator/2
  x/1 -> Bitwise Operator/1
  Bitwise Operator/1 -> Relational Operator/1

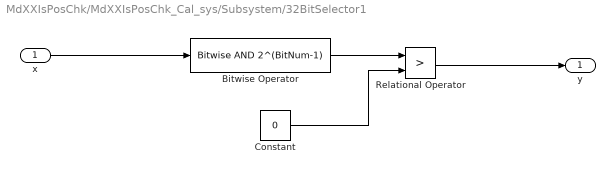
== system MdXXIsPosChk/MdXXIsPosChk_Cal_sys/Subsystem/32BitSelector1 ==
  x : Inport
  Bitwise Operator : simulink/Logic and Bit Operations/Bitwise Operator  logicop=AND  UseBitMask=on  BitMask=2^(BitNum-1)  BitMaskRealWorld=Stored Integer
  Constant : Constant  Value=0  OutDataTypeStr=uint32
  Relational Operator : RelationalOperator  Operator=>  OutDataTypeStr=boolean  RndMeth=Simplest  InputSameDT=off
  y : Outport  VectorParamsAs1DForOutWhenUnconnected=off
  wires:
  Bitwise Operator/1 -> Relational Operator/1
  x/1 -> Bitwise Operator/1
  Constant/1 -> Relational Operator/2
  Relational Operator/1 -> y/1

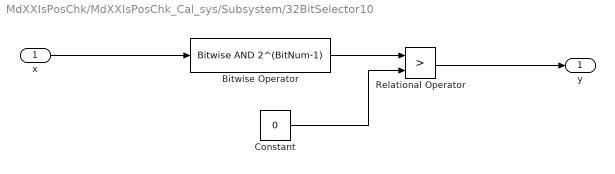
== system MdXXIsPosChk/MdXXIsPosChk_Cal_sys/Subsystem/32BitSelector10 ==
  x : Inport
  Bitwise Operator : simulink/Logic and Bit Operations/Bitwise Operator  logicop=AND  UseBitMask=on  BitMask=2^(BitNum-1)  BitMaskRealWorld=Stored Integer
  Constant : Constant  Value=0  OutDataTypeStr=uint32
  Relational Operator : RelationalOperator  Operator=>  OutDataTypeStr=boolean  RndMeth=Simplest  InputSameDT=off
  y : Outport  VectorParamsAs1DForOutWhenUnconnected=off
  wires:
  Bitwise Operator/1 -> Relational Operator/1
  x/1 -> Bitwise Operator/1
  Constant/1 -> Relational Operator/2
  Relational Operator/1 -> y/1

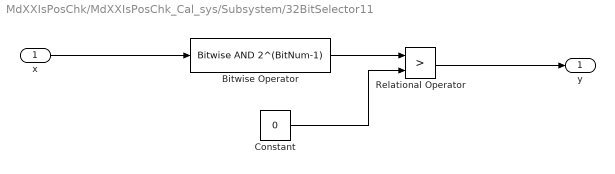
== system MdXXIsPosChk/MdXXIsPosChk_Cal_sys/Subsystem/32BitSelector11 ==
  x : Inport
  Bitwise Operator : simulink/Logic and Bit Operations/Bitwise Operator  logicop=AND  UseBitMask=on  BitMask=2^(BitNum-1)  BitMaskRealWorld=Stored Integer
  Constant : Constant  Value=0  OutDataTypeStr=uint32
  Relational Operator : RelationalOperator  Operator=>  OutDataTypeStr=boolean  RndMeth=Simplest  InputSameDT=off
  y : Outport  VectorParamsAs1DForOutWhenUnconnected=off
  wires:
  Relational Operator/1 -> y/1
  Constant/1 -> Relational Operator/2
  x/1 -> Bitwise Operator/1
  Bitwise Operator/1 -> Relational Operator/1

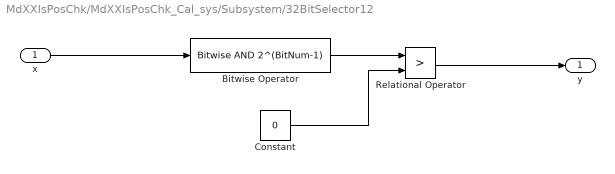
== system MdXXIsPosChk/MdXXIsPosChk_Cal_sys/Subsystem/32BitSelector12 ==
  x : Inport
  Bitwise Operator : simulink/Logic and Bit Operations/Bitwise Operator  logicop=AND  UseBitMask=on  BitMask=2^(BitNum-1)  BitMaskRealWorld=Stored Integer
  Constant : Constant  Value=0  OutDataTypeStr=uint32
  Relational Operator : RelationalOperator  Operator=>  OutDataTypeStr=boolean  RndMeth=Simplest  InputSameDT=off
  y : Outport  VectorParamsAs1DForOutWhenUnconnected=off
  wires:
  Bitwise Operator/1 -> Relational Operator/1
  x/1 -> Bitwise Operator/1
  Constant/1 -> Relational Operator/2
  Relational Operator/1 -> y/1

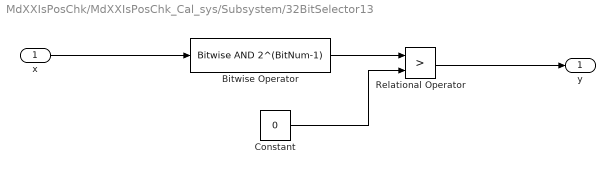
== system MdXXIsPosChk/MdXXIsPosChk_Cal_sys/Subsystem/32BitSelector13 ==
  x : Inport
  Bitwise Operator : simulink/Logic and Bit Operations/Bitwise Operator  logicop=AND  UseBitMask=on  BitMask=2^(BitNum-1)  BitMaskRealWorld=Stored Integer
  Constant : Constant  Value=0  OutDataTypeStr=uint32
  Relational Operator : RelationalOperator  Operator=>  OutDataTypeStr=boolean  RndMeth=Simplest  InputSameDT=off
  y : Outport  VectorParamsAs1DForOutWhenUnconnected=off
  wires:
  Relational Operator/1 -> y/1
  Constant/1 -> Relational Operator/2
  x/1 -> Bitwise Operator/1
  Bitwise Operator/1 -> Relational Operator/1

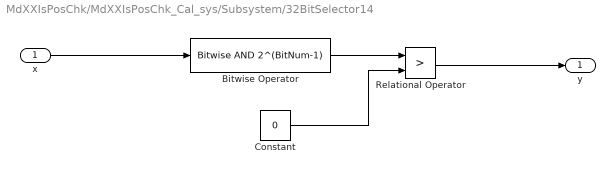
== system MdXXIsPosChk/MdXXIsPosChk_Cal_sys/Subsystem/32BitSelector14 ==
  x : Inport
  Bitwise Operator : simulink/Logic and Bit Operations/Bitwise Operator  logicop=AND  UseBitMask=on  BitMask=2^(BitNum-1)  BitMaskRealWorld=Stored Integer
  Constant : Constant  Value=0  OutDataTypeStr=uint32
  Relational Operator : RelationalOperator  Operator=>  OutDataTypeStr=boolean  RndMeth=Simplest  InputSameDT=off
  y : Outport  VectorParamsAs1DForOutWhenUnconnected=off
  wires:
  Relational Operator/1 -> y/1
  Constant/1 -> Relational Operator/2
  x/1 -> Bitwise Operator/1
  Bitwise Operator/1 -> Relational Operator/1

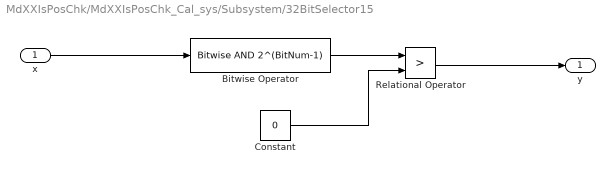
== system MdXXIsPosChk/MdXXIsPosChk_Cal_sys/Subsystem/32BitSelector15 ==
  x : Inport
  Bitwise Operator : simulink/Logic and Bit Operations/Bitwise Operator  logicop=AND  UseBitMask=on  BitMask=2^(BitNum-1)  BitMaskRealWorld=Stored Integer
  Constant : Constant  Value=0  OutDataTypeStr=uint32
  Relational Operator : RelationalOperator  Operator=>  OutDataTypeStr=boolean  RndMeth=Simplest  InputSameDT=off
  y : Outport  VectorParamsAs1DForOutWhenUnconnected=off
  wires:
  Bitwise Operator/1 -> Relational Operator/1
  x/1 -> Bitwise Operator/1
  Constant/1 -> Relational Operator/2
  Relational Operator/1 -> y/1

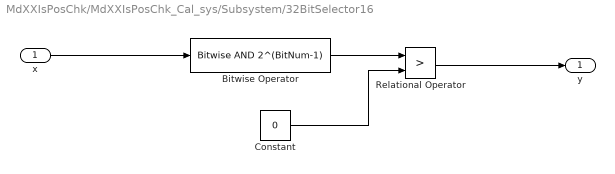
== system MdXXIsPosChk/MdXXIsPosChk_Cal_sys/Subsystem/32BitSelector16 ==
  x : Inport
  Bitwise Operator : simulink/Logic and Bit Operations/Bitwise Operator  logicop=AND  UseBitMask=on  BitMask=2^(BitNum-1)  BitMaskRealWorld=Stored Integer
  Constant : Constant  Value=0  OutDataTypeStr=uint32
  Relational Operator : RelationalOperator  Operator=>  OutDataTypeStr=boolean  RndMeth=Simplest  InputSameDT=off
  y : Outport  VectorParamsAs1DForOutWhenUnconnected=off
  wires:
  Relational Operator/1 -> y/1
  Constant/1 -> Relational Operator/2
  x/1 -> Bitwise Operator/1
  Bitwise Operator/1 -> Relational Operator/1

== system MdXXIsPosChk/MdXXIsPosChk_Cal_sys/Subsystem/32BitSelector17 ==
  x : Inport
  Bitwise Operator : simulink/Logic and Bit Operations/Bitwise Operator  logicop=AND  UseBitMask=on  BitMask=2^(BitNum-1)  BitMaskRealWorld=Stored Integer
  Constant : Constant  Value=0  OutDataTypeStr=uint32
  Relational Operator : RelationalOperator  Operator=>  OutDataTypeStr=boolean  RndMeth=Simplest  InputSameDT=off
  y : Outport  VectorParamsAs1DForOutWhenUnconnected=off
  wires:
  Bitwise Operator/1 -> Relational Operator/1
  x/1 -> Bitwise Operator/1
  Constant/1 -> Relational Operator/2
  Relational Operator/1 -> y/1

== system MdXXIsPosChk/MdXXIsPosChk_Cal_sys/Subsystem/32BitSelector18 ==
  x : Inport
  Bitwise Operator : simulink/Logic and Bit Operations/Bitwise Operator  logicop=AND  UseBitMask=on  BitMask=2^(BitNum-1)  BitMaskRealWorld=Stored Integer
  Constant : Constant  Value=0  OutDataTypeStr=uint32
  Relational Operator : RelationalOperator  Operator=>  OutDataTypeStr=boolean  RndMeth=Simplest  InputSameDT=off
  y : Outport  VectorParamsAs1DForOutWhenUnconnected=off
  wires:
  Relational Operator/1 -> y/1
  Constant/1 -> Relational Operator/2
  x/1 -> Bitwise Operator/1
  Bitwise Operator/1 -> Relational Operator/1

== system MdXXIsPosChk/MdXXIsPosChk_Cal_sys/Subsystem/32BitSelector19 ==
  x : Inport
  Bitwise Operator : simulink/Logic and Bit Operations/Bitwise Operator  logicop=AND  UseBitMask=on  BitMask=2^(BitNum-1)  BitMaskRealWorld=Stored Integer
  Constant : Constant  Value=0  OutDataTypeStr=uint32
  Relational Operator : RelationalOperator  Operator=>  OutDataTypeStr=boolean  RndMeth=Simplest  InputSameDT=off
  y : Outport  VectorParamsAs1DForOutWhenUnconnected=off
  wires:
  Bitwise Operator/1 -> Relational Operator/1
  x/1 -> Bitwise Operator/1
  Constant/1 -> Relational Operator/2
  Relational Operator/1 -> y/1

== system MdXXIsPosChk/MdXXIsPosChk_Cal_sys/Subsystem/32BitSelector2 ==
  x : Inport
  Bitwise Operator : simulink/Logic and Bit Operations/Bitwise Operator  logicop=AND  UseBitMask=on  BitMask=2^(BitNum-1)  BitMaskRealWorld=Stored Integer
  Constant : Constant  Value=0  OutDataTypeStr=uint32
  Relational Operator : RelationalOperator  Operator=>  OutDataTypeStr=boolean  RndMeth=Simplest  InputSameDT=off
  y : Outport  VectorParamsAs1DForOutWhenUnconnected=off
  wires:
  Bitwise Operator/1 -> Relational Operator/1
  x/1 -> Bitwise Operator/1
  Constant/1 -> Relational Operator/2
  Relational Operator/1 -> y/1

== system MdXXIsPosChk/MdXXIsPosChk_Cal_sys/Subsystem/32BitSelector3 ==
  x : Inport
  Bitwise Operator : simulink/Logic and Bit Operations/Bitwise Operator  logicop=AND  UseBitMask=on  BitMask=2^(BitNum-1)  BitMaskRealWorld=Stored Integer
  Constant : Constant  Value=0  OutDataTypeStr=uint32
  Relational Operator : RelationalOperator  Operator=>  OutDataTypeStr=boolean  RndMeth=Simplest  InputSameDT=off
  y : Outport  VectorParamsAs1DForOutWhenUnconnected=off
  wires:
  Relational Operator/1 -> y/1
  Constant/1 -> Relational Operator/2
  x/1 -> Bitwise Operator/1
  Bitwise Operator/1 -> Relational Operator/1

== system MdXXIsPosChk/MdXXIsPosChk_Cal_sys/Subsystem/32BitSelector4 ==
  x : Inport
  Bitwise Operator : simulink/Logic and Bit Operations/Bitwise Operator  logicop=AND  UseBitMask=on  BitMask=2^(BitNum-1)  BitMaskRealWorld=Stored Integer
  Constant : Constant  Value=0  OutDataTypeStr=uint32
  Relational Operator : RelationalOperator  Operator=>  OutDataTypeStr=boolean  RndMeth=Simplest  InputSameDT=off
  y : Outport  VectorParamsAs1DForOutWhenUnconnected=off
  wires:
  Bitwise Operator/1 -> Relational Operator/1
  x/1 -> Bitwise Operator/1
  Constant/1 -> Relational Operator/2
  Relational Operator/1 -> y/1

== system MdXXIsPosChk/MdXXIsPosChk_Cal_sys/Subsystem/32BitSelector5 ==
  x : Inport
  Bitwise Operator : simulink/Logic and Bit Operations/Bitwise Operator  logicop=AND  UseBitMask=on  BitMask=2^(BitNum-1)  BitMaskRealWorld=Stored Integer
  Constant : Constant  Value=0  OutDataTypeStr=uint32
  Relational Operator : RelationalOperator  Operator=>  OutDataTypeStr=boolean  RndMeth=Simplest  InputSameDT=off
  y : Outport  VectorParamsAs1DForOutWhenUnconnected=off
  wires:
  Relational Operator/1 -> y/1
  Constant/1 -> Relational Operator/2
  x/1 -> Bitwise Operator/1
  Bitwise Operator/1 -> Relational Operator/1

== system MdXXIsPosChk/MdXXIsPosChk_Cal_sys/Subsystem/32BitSelector6 ==
  x : Inport
  Bitwise Operator : simulink/Logic and Bit Operations/Bitwise Operator  logicop=AND  UseBitMask=on  BitMask=2^(BitNum-1)  BitMaskRealWorld=Stored Integer
  Constant : Constant  Value=0  OutDataTypeStr=uint32
  Relational Operator : RelationalOperator  Operator=>  OutDataTypeStr=boolean  RndMeth=Simplest  InputSameDT=off
  y : Outport  VectorParamsAs1DForOutWhenUnconnected=off
  wires:
  Relational Operator/1 -> y/1
  Constant/1 -> Relational Operator/2
  x/1 -> Bitwise Operator/1
  Bitwise Operator/1 -> Relational Operator/1

== system MdXXIsPosChk/MdXXIsPosChk_Cal_sys/Subsystem/32BitSelector7 ==
  x : Inport
  Bitwise Operator : simulink/Logic and Bit Operations/Bitwise Operator  logicop=AND  UseBitMask=on  BitMask=2^(BitNum-1)  BitMaskRealWorld=Stored Integer
  Constant : Constant  Value=0  OutDataTypeStr=uint32
  Relational Operator : RelationalOperator  Operator=>  OutDataTypeStr=boolean  RndMeth=Simplest  InputSameDT=off
  y : Outport  VectorParamsAs1DForOutWhenUnconnected=off
  wires:
  Bitwise Operator/1 -> Relational Operator/1
  x/1 -> Bitwise Operator/1
  Constant/1 -> Relational Operator/2
  Relational Operator/1 -> y/1

== system MdXXIsPosChk/MdXXIsPosChk_Cal_sys/Subsystem/32BitSelector8 ==
  x : Inport
  Bitwise Operator : simulink/Logic and Bit Operations/Bitwise Operator  logicop=AND  UseBitMask=on  BitMask=2^(BitNum-1)  BitMaskRealWorld=Stored Integer
  Constant : Constant  Value=0  OutDataTypeStr=uint32
  Relational Operator : RelationalOperator  Operator=>  OutDataTypeStr=boolean  RndMeth=Simplest  InputSameDT=off
  y : Outport  VectorParamsAs1DForOutWhenUnconnected=off
  wires:
  Relational Operator/1 -> y/1
  Constant/1 -> Relational Operator/2
  x/1 -> Bitwise Operator/1
  Bitwise Operator/1 -> Relational Operator/1

== system MdXXIsPosChk/MdXXIsPosChk_Cal_sys/Subsystem/32BitSelector9 ==
  x : Inport
  Bitwise Operator : simulink/Logic and Bit Operations/Bitwise Operator  logicop=AND  UseBitMask=on  BitMask=2^(BitNum-1)  BitMaskRealWorld=Stored Integer
  Constant : Constant  Value=0  OutDataTypeStr=uint32
  Relational Operator : RelationalOperator  Operator=>  OutDataTypeStr=boolean  RndMeth=Simplest  InputSameDT=off
  y : Outport  VectorParamsAs1DForOutWhenUnconnected=off
  wires:
  Bitwise Operator/1 -> Relational Operator/1
  x/1 -> Bitwise Operator/1
  Constant/1 -> Relational Operator/2
  Relational Operator/1 -> y/1
